simulink model "untitled"  (R2023b)
settings: Solver=VariableStepAuto  StartTime=0.0  StopTime=10.0  RelTol=1e-3
libraries: spsMosfetLib x6
settings Model: Creator=10166  LastModifiedBy=10166

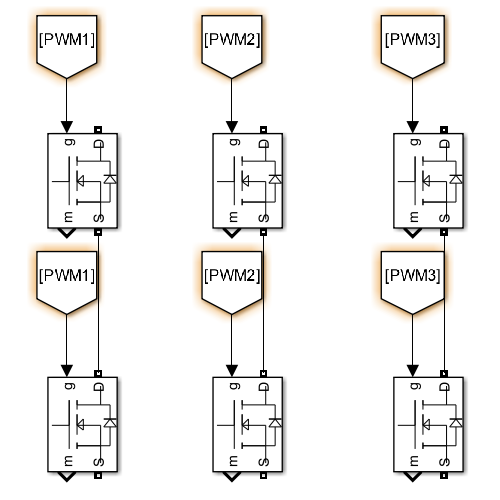
[thumbnail: Simulink's stored preview of the top-level diagram]
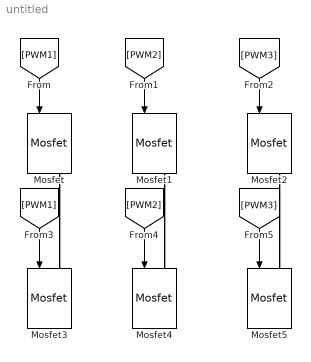
== system untitled ==
  Mosfet{,1..5} (6 alike) : spsMosfetLib/Mosfet  Ron=0.1  Lon=0  Rd=0.01  Vfd=0  IC=0  Rs=1e5  Cs=inf  Measurements=on
  wires:
  [PWM1] -> Mosfet/1
  [PWM2] -> Mosfet1/1
  [PWM3] -> Mosfet2/1
  [PWM1] -> Mosfet3/1
  [PWM2] -> Mosfet4/1
  [PWM3] -> Mosfet5/1
  connections:
  Mosfet/RConn1 -- Mosfet3/LConn1
  Mosfet1/RConn1 -- Mosfet4/LConn1
  Mosfet2/RConn1 -- Mosfet5/LConn1
